simulink model "simu5"  (R2021a)
settings: Solver=FixedStepAuto  StartTime=0.0  StopTime=60  FixedStep=0.001  RelTol=1e-3
libraries: cstblocks x10
settings Model: Creator=me-clab2  LastModifiedBy=HASEE
settings SolverCC: AlgebraicLoopSolver=TrustRegion
settings DebuggingCC: SFMachineParentedDataDiag=warning

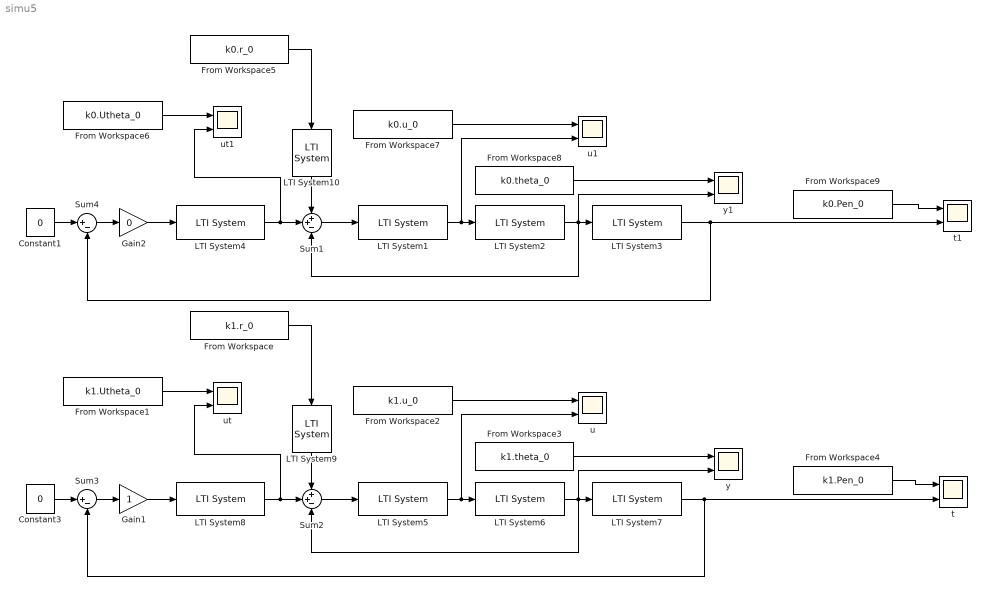
== system simu5 ==
  Constant1 : Constant  Value=0
  Constant3 : Constant  Value=0
  From Workspace : FromWorkspace  VariableName=k1.r_0  OutDataTypeStr=double
  From Workspace1 : FromWorkspace  VariableName=k1.Utheta_0  OutDataTypeStr=double
  From Workspace2 : FromWorkspace  VariableName=k1.u_0  OutDataTypeStr=double
  From Workspace3 : FromWorkspace  VariableName=k1.theta_0  OutDataTypeStr=double
  From Workspace4 : FromWorkspace  VariableName=k1.Pen_0  OutDataTypeStr=double
  From Workspace5 : FromWorkspace  VariableName=k0.r_0  OutDataTypeStr=double
  From Workspace6 : FromWorkspace  VariableName=k0.Utheta_0  OutDataTypeStr=double
  From Workspace7 : FromWorkspace  VariableName=k0.u_0  OutDataTypeStr=double
  From Workspace8 : FromWorkspace  VariableName=k0.theta_0  OutDataTypeStr=double
  From Workspace9 : FromWorkspace  VariableName=k0.Pen_0  OutDataTypeStr=double
  Gain1 : Gain
  Gain2 : Gain  Gain=0
  LTI System1 : cstblocks/LTI System  sys=Cy  IC=[]
  LTI System10 : cstblocks/LTI System  sys=F  IC=[]
  LTI System2 : cstblocks/LTI System  sys=Py  IC=[]
  LTI System3 : cstblocks/LTI System  sys=Pt  IC=[]
  LTI System4 : cstblocks/LTI System  sys=Ctheta  IC=[]
  LTI System5 : cstblocks/LTI System  sys=Cy  IC=[]
  LTI System6 : cstblocks/LTI System  sys=Py  IC=[]
  LTI System7 : cstblocks/LTI System  sys=Pt  IC=[]
  LTI System8 : cstblocks/LTI System  sys=Ctheta  IC=[]
  LTI System9 : cstblocks/LTI System  sys=F  IC=[]
  Sum1 : Sum  Inputs=++-
  Sum2 : Sum  Inputs=++-
  Sum3 : Sum  Inputs=|+-
  Sum4 : Sum  Inputs=|+-
  t : Scope  NumInputPorts=2
  t1 : Scope  NumInputPorts=2
  u : Scope  NumInputPorts=2
  u1 : Scope  NumInputPorts=2
  ut : Scope  NumInputPorts=2
  ut1 : Scope  NumInputPorts=2
  y : Scope  NumInputPorts=2
  y1 : Scope  NumInputPorts=2
  wires:
  Constant3/1 -> Sum3/1
  LTI System6/1 -> y/2, Sum2/3, LTI System7/1
  LTI System9/1 -> Sum2/1
  Gain1/1 -> LTI System8/1
  Sum3/1 -> Gain1/1
  LTI System5/1 -> u/2, LTI System6/1
  LTI System8/1 -> ut/2, Sum2/2
  Sum2/1 -> LTI System5/1
  LTI System7/1 -> Sum3/2, t/2
  From Workspace/1 -> LTI System9/1
  From Workspace1/1 -> ut/1
  From Workspace2/1 -> u/1
  From Workspace3/1 -> y/1
  From Workspace4/1 -> t/1
  From Workspace8/1 -> y1/1
  From Workspace7/1 -> u1/1
  From Workspace6/1 -> ut1/1
  LTI System3/1 -> t1/2, Sum4/2
  LTI System4/1 -> ut1/2, Sum1/2
  Sum1/1 -> LTI System1/1
  Gain2/1 -> LTI System4/1
  From Workspace5/1 -> LTI System10/1
  LTI System1/1 -> u1/2, LTI System2/1
  LTI System10/1 -> Sum1/1
  LTI System2/1 -> y1/2, Sum1/3, LTI System3/1
  Sum4/1 -> Gain2/1
  Constant1/1 -> Sum4/1
  From Workspace9/1 -> t1/1
